simulink model "vhs_fpga_rx_to_sdram_time_share_agc_cfo"  (Simulink 7.1)
settings: Solver=FixedStepDiscrete  SolverMode=SingleTasking  StartTime=0.0  StopTime=inf  RelTol=1e-3
values from neighbouring files (symbols this model uses):
  N_FB_RX_frame = 390    [OFDM_Parameter.mat]
  Nfft = 64    [OFDM_Parameter.mat]
  Nguard = 16    [OFDM_Parameter.mat]
  Nofdm = 130    [OFDM_Parameter.mat]
  Nskip = 8    [OFDM_Parameter.mat]
undefined symbols (not defined in the file or in its folder): Fs, Sincos_Bits, Sincos_Len, Theta_Bits
libraries: xbsIndex_r4 x366, vhsadac_common_ob_fpgalib_v1_2_0 x18, misc_tools_fpgalib_v1_0_0 x6, rffe_fpgalib_v1_1_0 x1, rtdex_fpgalib_v1_1_0 x1
(part 2 of 5)

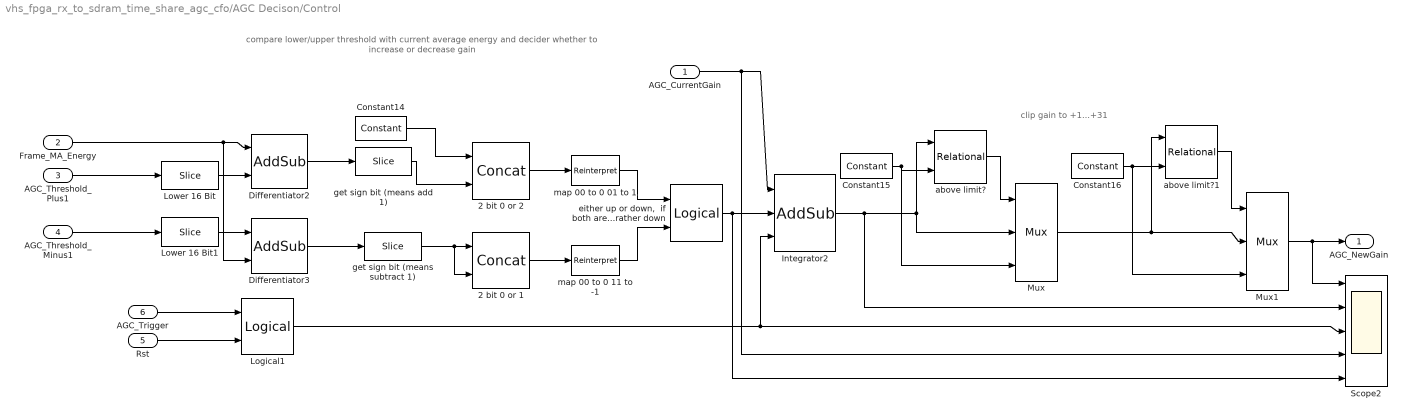
== system vhs_fpga_rx_to_sdram_time_share_agc_cfo/AGC Decison/Control ==
  note: compare lower/upper threshold with current average energy
      | and decider whether to increase or decrease gain
  note: clip gain to +1...+31
  AGC_CurrentGain : Inport
  Frame_MA_Energy : Inport  Port=2
  AGC_Threshold_Plus1 : Inport  Port=3
  AGC_Threshold_Minus1 : Inport  Port=4
  Rst : Inport  Port=5
  AGC_Trigger : Inport  Port=6
  2 bit 0 or 1 : xbsIndex_r4/Concat  num_inputs=2  dbl_ovrd=off  block_type=concat
      settings: block_version=10.1.3
  2 bit 0 or 2 : xbsIndex_r4/Concat  num_inputs=2  dbl_ovrd=off  block_type=concat
      settings: block_version=10.1.3
  Constant14 : xbsIndex_r4/Constant  arith_type=Unsigned  const=0  n_bits=1  bin_pt=0  explicit_period=on  period=5  equ=P=C  opselect=C  inp2=PCIN>>17  opr=+  inp1=P  carry=CIN  dbl_ovrd=off  block_type=constant
  Constant15 : xbsIndex_r4/Constant  arith_type=Signed (2's comp)  const=31  n_bits=32  bin_pt=0  explicit_period=on  period=5  equ=P=C  opselect=C  inp2=PCIN>>17  opr=+  inp1=P  carry=CIN  dbl_ovrd=off  block_type=constant
  Constant16 : xbsIndex_r4/Constant  arith_type=Signed (2's comp)  const=1  n_bits=32  bin_pt=0  explicit_period=on  period=5  equ=P=C  opselect=C  inp2=PCIN>>17  opr=+  inp1=P  carry=CIN  dbl_ovrd=off  block_type=constant
  Differentiator2 : xbsIndex_r4/AddSub  mode=Subtraction  use_carryin=off  use_carryout=off  en=off  latency=0  precision=Full  arith_type=Unsigned  n_bits=16  bin_pt=14  quantization=Truncate  overflow=Wrap  dbl_ovrd=off  use_behavioral_HDL=off  pipelined=off  use_rpm=on  hw_selection=Fabric  block_type=addsub
      settings: block_version=10.1.3
  Differentiator3 : xbsIndex_r4/AddSub  mode=Subtraction  use_carryin=off  use_carryout=off  en=off  latency=0  precision=Full  arith_type=Unsigned  n_bits=16  bin_pt=14  quantization=Truncate  overflow=Wrap  dbl_ovrd=off  use_behavioral_HDL=off  pipelined=off  use_rpm=on  hw_selection=Fabric  block_type=addsub
      settings: block_version=10.1.3
  Integrator2 : xbsIndex_r4/AddSub  mode=Addition  use_carryin=off  use_carryout=off  en=on  latency=1  precision=User Defined  arith_type="Signed  (2's comp)"  n_bits=32  bin_pt=0  quantization=Truncate  overflow=Saturate  dbl_ovrd=off  use_behavioral_HDL=off  pipelined=off  use_rpm=on  hw_selection=Fabric  block_type=addsub
      settings: block_version=10.1.3
  Logical1 : xbsIndex_r4/Logical  logical_function=OR  inputs=2  en=off  latency=0  precision=Full  arith_type=Unsigned  n_bits=16  bin_pt=0  align_bp=on  dbl_ovrd=off  block_type=logical
  Lower 16 Bit : xbsIndex_r4/Slice  nbits=16  boolean_output=off  mode=Upper Bit Location + Width  bit1=-16  base1=MSB of Input  bit0=0  base0=LSB of Input  dbl_ovrd=off  block_type=slice
      settings: infoedit="Extracts a given range of bits from each input sample and presents it at the output.  The output type is ordinarily unsigned with binary point at zero, but can be Boolean when the slice is one bit wide.<P><P>Hardware notes: In hardware this block costs nothing."  block_version=10.1.3
  Lower 16 Bit1 : xbsIndex_r4/Slice  nbits=16  boolean_output=off  mode=Upper Bit Location + Width  bit1=-16  base1=MSB of Input  bit0=0  base0=LSB of Input  dbl_ovrd=off  block_type=slice
      settings: infoedit="Extracts a given range of bits from each input sample and presents it at the output.  The output type is ordinarily unsigned with binary point at zero, but can be Boolean when the slice is one bit wide.<P><P>Hardware notes: In hardware this block costs nothing."  block_version=10.1.3
  Mux : xbsIndex_r4/Mux  inputs=2  en=off  latency=0  precision=Full  arith_type=Unsigned  n_bits=16  bin_pt=14  quantization=Truncate  overflow=Wrap  dbl_ovrd=off  block_type=mux
  Mux1 : xbsIndex_r4/Mux  inputs=2  en=off  latency=0  precision=Full  arith_type=Unsigned  n_bits=16  bin_pt=14  quantization=Truncate  overflow=Wrap  dbl_ovrd=off  block_type=mux
  Scope2 : Scope  NumInputPorts=5
      settings: TimeRange=369.8207656148967  YMin=1~0~0~0~0  YMax=2~2~1~15~1  SaveName=ScopeData2  MaxDataPoints=500000
  above limit? : xbsIndex_r4/Relational  mode=a>=b  en=off  latency=0  dbl_ovrd=off  block_type=relational
      settings: block_version=10.1.3
  above limit?1 : xbsIndex_r4/Relational  mode=a<=b  en=off  latency=0  dbl_ovrd=off  block_type=relational
      settings: block_version=10.1.3
  "either up or down,  if both are set, then rather down" : xbsIndex_r4/Logical  logical_function=OR  inputs=2  en=off  latency=0  precision=Full  arith_type=Unsigned  n_bits=16  bin_pt=0  align_bp=on  dbl_ovrd=off  block_type=logical
  get sign bit (means add 1) : xbsIndex_r4/Slice  nbits=1  boolean_output=off  mode=Upper Bit Location + Width  bit1=0  base1=MSB of Input  bit0=0  base0=LSB of Input  dbl_ovrd=off  block_type=slice
      settings: infoedit="Extracts a given range of bits from each input sample and presents it at the output.  The output type is ordinarily unsigned with binary point at zero, but can be Boolean when the slice is one bit wide.<P><P>Hardware notes: In hardware this block costs nothing."  block_version=10.1.3
  get sign bit (means subtract 1) : xbsIndex_r4/Slice  nbits=1  boolean_output=off  mode=Upper Bit Location + Width  bit1=0  base1=MSB of Input  bit0=0  base0=LSB of Input  dbl_ovrd=off  block_type=slice
      settings: infoedit="Extracts a given range of bits from each input sample and presents it at the output.  The output type is ordinarily unsigned with binary point at zero, but can be Boolean when the slice is one bit wide.<P><P>Hardware notes: In hardware this block costs nothing."  block_version=10.1.3
  map 00 to 0 01 to 1 : xbsIndex_r4/Reinterpret  force_arith_type=on  arith_type="Signed  (2's comp)"  force_bin_pt=on  bin_pt=0  block_type=reinterpret
      settings: infoedit="Changes signal type without altering the binary representation.   You can changed the signal between signed and unsigned, and relocate the binary point.<P><P>Hardware notes: In hardware this block costs nothing.<P><P>Example:  Suppose the input is 6 bits wide, signed, with 2 fractional bits, and the output is forced to unsigned with 0 fractional bits.  Then an input of -2.0 (1110.00 in binary 2's complement) becomes an output of 56 (111000 in binary)."  block_version=10.1.3
  map 00 to 0 11 to -1 : xbsIndex_r4/Reinterpret  force_arith_type=on  arith_type="Signed  (2's comp)"  force_bin_pt=on  bin_pt=0  block_type=reinterpret
      settings: infoedit="Changes signal type without altering the binary representation.   You can changed the signal between signed and unsigned, and relocate the binary point.<P><P>Hardware notes: In hardware this block costs nothing.<P><P>Example:  Suppose the input is 6 bits wide, signed, with 2 fractional bits, and the output is forced to unsigned with 0 fractional bits.  Then an input of -2.0 (1110.00 in binary 2's complement) becomes an output of 56 (111000 in binary)."  block_version=10.1.3
  AGC_NewGain : Outport
  wires:
  Lower 16 Bit/1 -> Differentiator2/2
  Frame_MA_Energy/1 -> Differentiator3/2, Differentiator2/1
  Lower 16 Bit1/1 -> Differentiator3/1
  Differentiator2/1 -> get sign bit (means add 1)/1
  Differentiator3/1 -> get sign bit (means subtract 1)/1
  get sign bit (means subtract 1)/1 -> 2 bit 0 or 1/1, 2 bit 0 or 1/2
  2 bit 0 or 1/1 -> map 00 to 0 11 to -1/1
  get sign bit (means add 1)/1 -> 2 bit 0 or 2/2
  Constant14/1 -> 2 bit 0 or 2/1
  2 bit 0 or 2/1 -> map 00 to 0 01 to 1/1
  map 00 to 0 01 to 1/1 -> "either up or down,  if both are set, then rather down"/1
  map 00 to 0 11 to -1/1 -> "either up or down,  if both are set, then rather down"/2
  "either up or down,  if both are set, then rather down"/1 -> Integrator2/2, Scope2/5
  Constant15/1 -> above limit?/2, Mux/3
  above limit?/1 -> Mux/1
  Integrator2/1 -> above limit?/1, Mux/2, Scope2/2
  Constant16/1 -> above limit?1/2, Mux1/3
  above limit?1/1 -> Mux1/1
  Mux1/1 -> Scope2/1, AGC_NewGain/1
  Mux/1 -> Mux1/2, above limit?1/1
  AGC_CurrentGain/1 -> Scope2/4, Integrator2/1
  AGC_Trigger/1 -> Logical1/1
  Logical1/1 -> Integrator2/3, Scope2/3
  AGC_Threshold_Plus1/1 -> Lower 16 Bit/1
  AGC_Threshold_Minus1/1 -> Lower 16 Bit1/1
  Rst/1 -> Logical1/2

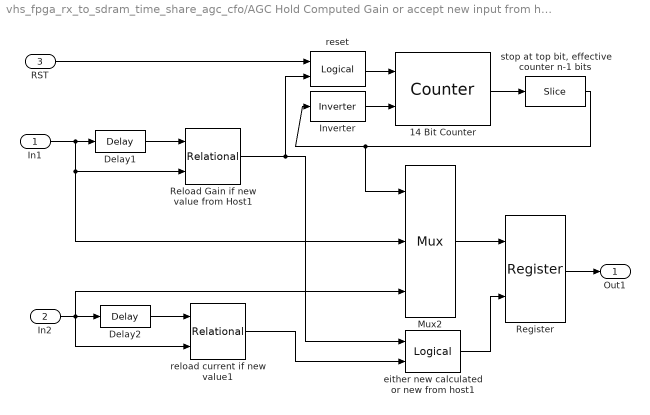
== system vhs_fpga_rx_to_sdram_time_share_agc_cfo/AGC Hold Computed Gain or accept new input from host ==
  In1 : Inport
  In2 : Inport  Port=2
  RST : Inport  Port=3
  14 Bit Counter : xbsIndex_r4/Counter  cnt_type=Free Running  cnt_to=Inf  operation=Up  start_count=0  cnt_by_val=1  arith_type=Unsigned  n_bits=14  bin_pt=0  load_pin=off  rst=on  en=on  explicit_period=off  period=1  dbl_ovrd=off  use_behavioral_HDL=off  use_rpm=off  implementation=Fabric  block_type=counter
  Delay1 : xbsIndex_r4/Delay  en=off  latency=1  dbl_ovrd=off  reg_retiming=off  block_type=delay
  Delay2 : xbsIndex_r4/Delay  en=off  latency=1  dbl_ovrd=off  reg_retiming=off  block_type=delay
  Inverter : xbsIndex_r4/Inverter  en=off  latency=0  dbl_ovrd=off  block_type=inv
  Mux2 : xbsIndex_r4/Mux  inputs=2  en=off  latency=0  precision=Full  arith_type=Unsigned  n_bits=16  bin_pt=14  quantization=Truncate  overflow=Wrap  dbl_ovrd=off  block_type=mux
  Register : xbsIndex_r4/Register  init=12  rst=off  en=on  dbl_ovrd=off  block_type=register
  Reload Gain if new value from Host1 : xbsIndex_r4/Relational  mode=a!=b  en=off  latency=1  dbl_ovrd=off  block_type=relational
      settings: block_version=10.1.3
  either new calculated or new from host1 : xbsIndex_r4/Logical  logical_function=OR  inputs=2  en=off  latency=1  precision=Full  arith_type=Unsigned  n_bits=16  bin_pt=0  align_bp=on  dbl_ovrd=off  block_type=logical
  reload current if new value1 : xbsIndex_r4/Relational  mode=a!=b  en=off  latency=1  dbl_ovrd=off  block_type=relational
      settings: block_version=10.1.3
  reset : xbsIndex_r4/Logical  logical_function=OR  inputs=2  en=off  latency=0  precision=Full  arith_type=Unsigned  n_bits=16  bin_pt=0  align_bp=on  dbl_ovrd=off  block_type=logical
  "stop at top bit, effective counter n-1 bits" : xbsIndex_r4/Slice  nbits=1  boolean_output=on  mode=Upper Bit Location + Width  bit1=0  base1=MSB of Input  bit0=0  base0=LSB of Input  dbl_ovrd=off  block_type=slice
      settings: infoedit="Extracts a given range of bits from each input sample and presents it at the output.  The output type is ordinarily unsigned with binary point at zero, but can be Boolean when the slice is one bit wide.<P><P>Hardware notes: In hardware this block costs nothing."  block_version=10.1.3
  Out1 : Outport
  wires:
  Delay1/1 -> Reload Gain if new value from Host1/1
  Reload Gain if new value from Host1/1 -> either new calculated or new from host1/1, reset/2
  Mux2/1 -> Register/1
  In1/1 -> Delay1/1, Reload Gain if new value from Host1/2, Mux2/2
  either new calculated or new from host1/1 -> Register/2
  Delay2/1 -> reload current if new value1/1
  In2/1 -> Delay2/1, reload current if new value1/2, Mux2/3
  reload current if new value1/1 -> either new calculated or new from host1/2
  Register/1 -> Out1/1
  Inverter/1 -> 14 Bit Counter/2
  "stop at top bit, effective counter n-1 bits"/1 -> Inverter/1, Mux2/1
  14 Bit Counter/1 -> "stop at top bit, effective counter n-1 bits"/1
  reset/1 -> 14 Bit Counter/1
  RST/1 -> reset/1

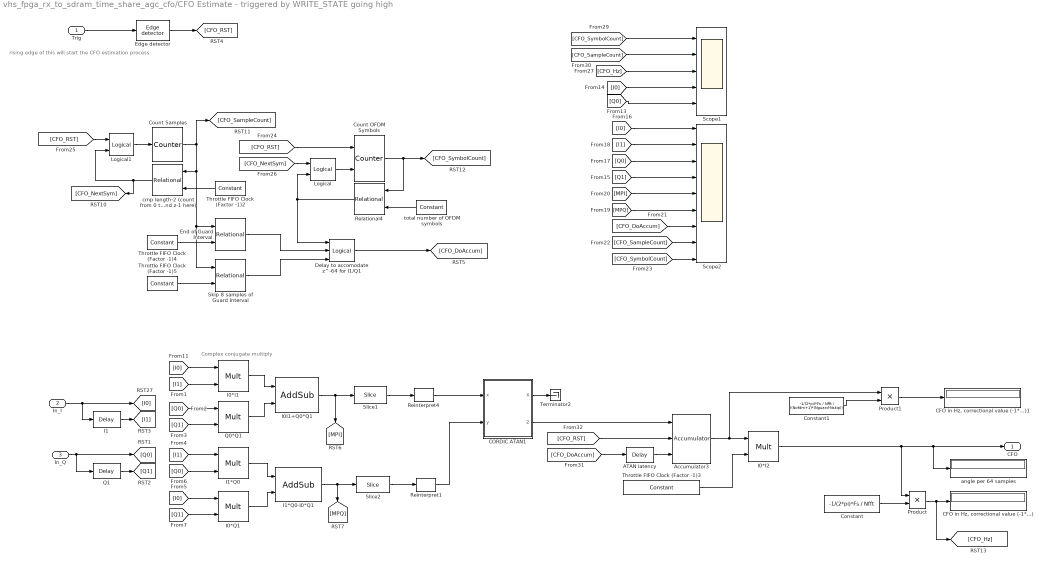
== system vhs_fpga_rx_to_sdram_time_share_agc_cfo/CFO Estimate - triggered by WRITE_STATE going high ==
  note: rising edge of this will start the
      | CFO estimation process
  note: Complex conjugate multiply
  Trig : Inport
  In_I : Inport  Port=2
  In_Q : Inport  Port=3
  ATAN latency : xbsIndex_r4/Delay  en=off  latency=16  dbl_ovrd=off  reg_retiming=off  block_type=delay
  Accumulator3 : xbsIndex_r4/Accumulator  operation=Add  n_bits=42  overflow=Saturate  scale=1  rst=on  hasbypass=off  en=on  dbl_ovrd=off  use_behavioral_HDL=on  implementation=Fabric  block_type=accum
      settings: infoedit="Adder or subtractor-based accumulator.   Output type and binary point position match the input.<P><P>Hardware notes: When \"Reinitialize with input 'b' on reset\" is selected, the accumulator is forced to run at the system rate even if the input 'b' is running at a slower rate."  block_version=10.1.3
  "CFO in Hz, correctional value (-1*...)" : Display
  "CFO in Hz, correctional value (-1*...)1" : Display
  CORDIC ATAN1 : Subsystem  mask(Xilinx CORDIC ATAN){stages=13, pe_nbits=32, pe_binpt=30, pipeline_x=ones(1,14), prev_stages=13, pipeline=[1  1  1  1  1  1  1  1  1  1  1  1  1]}
      mask prompts: stages "Number of Processing Elements (integer value starting from 1)"; pe_nbits "X, Y Data Width"; pe_binpt "X, Y Binary Point Position"; pipeline_x "Latency for each Processing Element [1 0 0 1]"; prev_stages "Previous Number of Stages"; pipeline "Previous Pipeline Values"
      mask help: A parallel implementation, circular vectoring mode CORDIC processor for performing rectangular-to-polar conversion. The number of iteration stages (and resultant output accuracy) and the processor arithmetic precision are controlled by the mask customization.
      mask init:
      | [bg,fg] = xlcmap('XBlock',0);
      | iPos = get_param(gcb,'Position');
      | iWidth=iPos(3)-iPos(1); iHeight=iPos(4)-iPos(2);
      | iCx=iWidth/2;
      | iCy=iHeight/2;
      | [logoX, logoY] = xlogo(iPos);
      | sav_gcb=gcb;
      | stages = round(sum(abs(stages)));
      | if (stages == 0)
      | 	stages = prev_stages;
      | end
      | x = zeros(1,stages);
      | pipe_size = max(size(pipeline_x));
      | if pipe_size >= stages
      | 	x(1,1:stages) = pipeline_x(1,1:stages);
      | else
      | 	x(1,1:pipe_size) = pipeline_x(1,1:pipe_size);
      | end
      | 
      | if (stages ~=prev_stages)
      | 	pipeline=x;
      | 	cordic_pe = find_system(gcb, 'lookUnderMasks', 'all', 'FollowLinks','on','masktype', 'CORDIC parallel PE');
      |     
      |   a=find_system(cordic_pe{1}, 'lookUnderMasks', 'all', 'FollowLinks','on','masktype', 'CORDIC iteration PE');
      |   for i= 2:length(a)
      |     for j=1:3
      | 	  delete_line(cordic_pe{1}, ['CORDIC PE' int2str(i-1) '/' int2str(j)], ['CORDIC PE' int2str(i) '/' int2str(j)]);
      |     end
      |   end
      |     if length(a)>0,
      |       delete_line(cordic_pe{1}, 'x/1', 'CORDIC PE1/1');
      |       delete_line(cordic_pe{1}, 'y/1', 'CORDIC PE1/2');
      |       delete_line(cordic_pe{1}, 'z/1', 'CORDIC PE1/3');
      |       delete_line(cordic_pe{1}, ['CORDIC PE' int2str(length(a)) '/1'],'X/1');
      |       delete_line(cordic_pe{1}, ['CORDIC PE' int2str(length(a)) '/2'],'Terminator/1');
      |       delete_line(cordic_pe{1}, ['CORDIC PE' int2str(length(a)) '/3'],'Z/1');
      |     elseif length(a)==0
      |       temp_port=get_param([cordic_pe{1} '/x'],'porthandles');
      |       temp_line=get_param(temp_port.Outport,'line');
      |       if temp_line>=0  delete_line(temp_line); end
      |       temp_port=get_param([cordic_pe{1} '/y'],'porthandles');
      |       temp_line=get_param(temp_port.Outport,'line');
      |       if temp_line>=0  delete_line(temp_line); end
      |       temp_port=get_param([cordic_pe{1} '/z'],'porthandles');
      |       temp_line=get_param(temp_port.Outport,'line');
      |       if temp_line>=0  delete_line(temp_line); end
      |     end
      | 
      |     for i=2:length(a)
      |       delete_block(a{i});
      |     end
      |     for i=2:stages,
      |         add_block([cordic_pe{1} '/CORDIC PE1'], [cordic_pe{1} '/CORDIC PE' int2str(i)], 'ii', int2str(i-1),'pe_nbits', 'pe_nbits','pe_binpt', 'pe_binpt','pipeline',['pipeline(1,' int2str(i) ')'],'position',[150+(i-1)*125, 70, 205+(i-1)*125, 130]);
      |     end
      | 
      |     for i= 2:stages,
      |       for j=1:3
      | 		add_line(cordic_pe{1}, ['CORDIC PE' int2str(i-1) '/' int2str(j)], ['CORDIC PE' int2str(i) '/' int2str(j)], 'autorouting', 'on');
      |       end
      |     end
      | 
      |     if stages==0
      |       add_line(cordic_pe{1}, 'x/1', 'X/1', 'autorouting', 'on');
      |       add_line(cordic_pe{1}, 'y/1', 'Terminator/1', 'autorouting', 'on');
      |       add_line(cordic_pe{1}, 'z/1', 'Z/1', 'autorouting', 'on');
      |     elseif stages>0
      |       add_line(cordic_pe{1}, 'x/1', 'CORDIC PE1/1', 'autorouting', 'on');
      |       add_line(cordic_pe{1}, 'y/1', 'CORDIC PE1/2', 'autorouting', 'on');
      |       add_line(cordic_pe{1}, 'z/1', 'CORDIC PE1/3', 'autorouting', 'on');
      | 
      |       set_param([cordic_pe{1} '/' 'X'], 'Position', [150+stages*125, 72, 180+stages*125, 86]);
      |       set_param([cordic_pe{1} '/' 'Terminator'], 'Position', [210+stages*125, 92, 225+stages*125, 108]);
      |       set_param([cordic_pe{1} '/' 'Z'], 'Position', [240+stages*125, 113, 270+stages*125, 127]);
      | 
      |       add_line(cordic_pe{1}, ['CORDIC PE' int2str(stages) '/1'], 'X/1', 'autorouting', 'on');
      |       add_line(cordic_pe{1}, ['CORDIC PE' int2str(stages) '/2'], 'Terminator/1', 'autorouting', 'on');
      |       add_line(cordic_pe{1}, ['CORDIC PE' int2str(stages) '/3'],'Z/1', 'autorouting', 'on');
      | 
      |       % force a "compile" of the constituent constant blocks to
      |       % workaround a data propagation problem
      |       find_system(cordic_pe{1}, 'lookUnderMasks', 'all', 'FollowLinks', 'on', 'MaskType','Xilinx Constant Block');
      |   end
      | 	set_param(sav_gcb, 'prev_stages', int2str(stages));
      | 	set_param(sav_gcb, 'pipeline', [ '[' int2str(x) ']']);
      | else
      | 	if (sum(pipeline~=x))
      | 		set_param(gcb, 'pipeline', [ '[' int2str(x) ']']);
      | 	end
      | end
      | str = sprintf('-%d',sum(x) + 3);
      settings: CopyFcn=set_param(gcb, 'MaskSelfModifiable', 'on', 'LinkStatus', 'none');
      mask Help: eval('');xlDoc('-book','sysgen','-topic','CORDIC_ATAN');
      mask Display:
      | patch([0 iWidth iWidth 0],[0 0 iHeight iHeight] , bg);
      | patch(logoX,logoY , fg);
      | text(iCx-6,iCy,'z');
      | text(iCx,iCy+4,str);
      | port_label('input',1,'x');
      | port_label('input',2,'y');
      | port_label('output',1,'mag');
      | port_label('output',2,'atan');
      | plot([0 0 iWidth iWidth 0], [0 iHeight iHeight 0 0]);
  Constant : Constant  Value=-1/(2*pi)*Fs / Nfft  OutDataType=sfix(16)  OutScaling=2^0  SampleTime=5
  Constant1 : Constant  Value=-1/(2*pi)*Fs / Nfft / ((Nofdm+1)*(Nguard-Nskip))  OutDataType=sfix(16)  OutScaling=2^0  SampleTime=5
  Count Samples : xbsIndex_r4/Counter  cnt_type=Free Running  cnt_to=Inf  operation=Up  start_count=0  cnt_by_val=1  arith_type=Unsigned  n_bits=7  bin_pt=0  load_pin=off  rst=on  en=off  explicit_period=on  period=5  dbl_ovrd=off  use_behavioral_HDL=off  use_rpm=off  implementation=Fabric  block_type=counter
      settings: block_version=VER_STRING_GOES_HERE
  Count OFDM Symbols : xbsIndex_r4/Counter  cnt_type=Free Running  cnt_to=Inf  operation=Up  start_count=0  cnt_by_val=1  arith_type=Unsigned  n_bits=8  bin_pt=0  load_pin=off  rst=on  en=on  explicit_period=on  period=5  dbl_ovrd=off  use_behavioral_HDL=off  use_rpm=off  implementation=Fabric  block_type=counter
      settings: block_version=VER_STRING_GOES_HERE
  Delay to accomodate z^-64 for I1/Q1 : xbsIndex_r4/Logical  logical_function=AND  inputs=3  en=off  latency=Nfft-3+1  precision=Full  arith_type=Unsigned  n_bits=16  bin_pt=0  align_bp=on  dbl_ovrd=off  block_type=logical
  Edge detector : misc_tools_fpgalib_v1_0_0/Edge detector  Tag=LYR_FPGA_MISC_EDGE_DETECTOR  Description=Lyrtech block  SystemSampleTime=-1  edge_detect=Rising  and_latency=0
  End of Guard Interval : xbsIndex_r4/Relational  mode=a<=b  en=off  latency=0  dbl_ovrd=off  block_type=relational
      settings: block_version=VER_STRING_GOES_HERE
  I0*I1 : xbsIndex_r4/Mult  precision=Full  arith_type="Signed  (2's comp)"  n_bits=16  bin_pt=14  quantization=Truncate  overflow=Wrap  en=off  latency=3  dbl_ovrd=off  use_behavioral_HDL=off  use_embedded=on  opt=Speed  optimum_pipeline=off  pipeline=on  use_rpm=on  placement_style=Triangular  block_type=mult
      settings: infoedit=Hardware notes: To use the internal pipeline stage of the dedicated multiplier you must select 'Pipeline for maximum performance'.  block_version=10.1.3
  I0*I2 : xbsIndex_r4/Mult  precision=User Defined  arith_type="Signed  (2's comp)"  n_bits=32  bin_pt=30  quantization=Truncate  overflow=Wrap  en=off  latency=3  dbl_ovrd=off  use_behavioral_HDL=off  use_embedded=on  opt=Speed  optimum_pipeline=off  pipeline=on  use_rpm=on  placement_style=Triangular  block_type=mult
      settings: infoedit=Hardware notes: To use the internal pipeline stage of the dedicated multiplier you must select 'Pipeline for maximum performance'.  block_version=10.1.3
  I0*Q1 : xbsIndex_r4/Mult  precision=Full  arith_type="Signed  (2's comp)"  n_bits=16  bin_pt=14  quantization=Truncate  overflow=Wrap  en=off  latency=3  dbl_ovrd=off  use_behavioral_HDL=off  use_embedded=on  opt=Speed  optimum_pipeline=off  pipeline=on  use_rpm=on  placement_style=Triangular  block_type=mult
      settings: infoedit=Hardware notes: To use the internal pipeline stage of the dedicated multiplier you must select 'Pipeline for maximum performance'.  block_version=10.1.3
  I0I1+Q0*Q1 : xbsIndex_r4/AddSub  mode=Addition  use_carryin=off  use_carryout=off  en=off  latency=1  precision=Full  arith_type=Unsigned  n_bits=16  bin_pt=14  quantization=Truncate  overflow=Wrap  dbl_ovrd=off  use_behavioral_HDL=off  pipelined=off  use_rpm=on  hw_selection=Fabric  block_type=addsub
      settings: block_version=10.1.3
  I1 : xbsIndex_r4/Delay  en=off  latency=Nfft  dbl_ovrd=off  reg_retiming=off  block_type=delay
  I1*Q0 : xbsIndex_r4/Mult  precision=Full  arith_type="Signed  (2's comp)"  n_bits=16  bin_pt=14  quantization=Truncate  overflow=Wrap  en=off  latency=3  dbl_ovrd=off  use_behavioral_HDL=off  use_embedded=on  opt=Speed  optimum_pipeline=off  pipeline=on  use_rpm=on  placement_style=Triangular  block_type=mult
      settings: infoedit=Hardware notes: To use the internal pipeline stage of the dedicated multiplier you must select 'Pipeline for maximum performance'.  block_version=10.1.3
  I1*Q0-I0*Q1 : xbsIndex_r4/AddSub  mode=Subtraction  use_carryin=off  use_carryout=off  en=off  latency=1  precision=Full  arith_type=Unsigned  n_bits=16  bin_pt=14  quantization=Truncate  overflow=Wrap  dbl_ovrd=off  use_behavioral_HDL=off  pipelined=off  use_rpm=on  hw_selection=Fabric  block_type=addsub
      settings: block_version=10.1.3
  Logical : xbsIndex_r4/Logical  logical_function=AND  inputs=2  en=off  latency=0  precision=Full  arith_type=Unsigned  n_bits=16  bin_pt=0  align_bp=on  dbl_ovrd=off  block_type=logical
  Logical1 : xbsIndex_r4/Logical  logical_function=OR  inputs=2  en=off  latency=0  precision=Full  arith_type=Unsigned  n_bits=16  bin_pt=0  align_bp=on  dbl_ovrd=off  block_type=logical
  Product : Product  OutDataType=sfix(16)  OutScaling=2^0  RndMeth=Zero
  Product1 : Product  OutDataType=sfix(16)  OutScaling=2^0  RndMeth=Zero
  Q0*Q1 : xbsIndex_r4/Mult  precision=Full  arith_type="Signed  (2's comp)"  n_bits=16  bin_pt=14  quantization=Truncate  overflow=Wrap  en=off  latency=3  dbl_ovrd=off  use_behavioral_HDL=off  use_embedded=on  opt=Speed  optimum_pipeline=off  pipeline=on  use_rpm=on  placement_style=Triangular  block_type=mult
      settings: infoedit=Hardware notes: To use the internal pipeline stage of the dedicated multiplier you must select 'Pipeline for maximum performance'.  block_version=10.1.3
  Q1 : xbsIndex_r4/Delay  en=off  latency=Nfft  dbl_ovrd=off  reg_retiming=off  block_type=delay
  Reinterpret1 : xbsIndex_r4/Reinterpret  force_arith_type=on  arith_type="Signed  (2's comp)"  force_bin_pt=on  bin_pt=30  block_type=reinterpret
      settings: infoedit="Changes signal type without altering the binary representation.   You can changed the signal between signed and unsigned, and relocate the binary point.<P><P>Hardware notes: In hardware this block costs nothing.<P><P>Example:  Suppose the input is 6 bits wide, signed, with 2 fractional bits, and the output is forced to unsigned with 0 fractional bits.  Then an input of -2.0 (1110.00 in binary 2's complement) becomes an output of 56 (111000 in binary)."  block_version=10.1.3
  Reinterpret4 : xbsIndex_r4/Reinterpret  force_arith_type=on  arith_type="Signed  (2's comp)"  force_bin_pt=on  bin_pt=30  block_type=reinterpret
      settings: infoedit="Changes signal type without altering the binary representation.   You can changed the signal between signed and unsigned, and relocate the binary point.<P><P>Hardware notes: In hardware this block costs nothing.<P><P>Example:  Suppose the input is 6 bits wide, signed, with 2 fractional bits, and the output is forced to unsigned with 0 fractional bits.  Then an input of -2.0 (1110.00 in binary 2's complement) becomes an output of 56 (111000 in binary)."  block_version=10.1.3
  Relational4 : xbsIndex_r4/Relational  Orientation=left  mode=a<b  en=off  latency=0  dbl_ovrd=off  block_type=relational
      settings: block_version=VER_STRING_GOES_HERE
  Scope1 : Scope  NumInputPorts=5
      settings: YMin=-5~-5~-5~-5~-5  YMax=5~5~5~5~5  SaveName=ScopeData8  MaxDataPoints=500000
  Scope2 : Scope  NumInputPorts=9
      settings: YMin=-5~-5~-5~-5~-5~-5~-5~-5~-5  YMax=5~5~5~5~5~5~5~5~5  MaxDataPoints=500000
  Skip 8 samples of Guard Interval : xbsIndex_r4/Relational  mode=a>b  en=off  latency=0  dbl_ovrd=off  block_type=relational
      settings: block_version=VER_STRING_GOES_HERE
  Slice1 : xbsIndex_r4/Slice  nbits=32  boolean_output=off  mode=Upper Bit Location + Width  bit1=0  base1=MSB of Input  bit0=0  base0=LSB of Input  dbl_ovrd=off  block_type=slice
      settings: infoedit="Extracts a given range of bits from each input sample and presents it at the output.  The output type is ordinarily unsigned with binary point at zero, but can be Boolean when the slice is one bit wide.<P><P>Hardware notes: In hardware this block costs nothing."  block_version=10.1.3
  Slice2 : xbsIndex_r4/Slice  nbits=32  boolean_output=off  mode=Upper Bit Location + Width  bit1=0  base1=MSB of Input  bit0=0  base0=LSB of Input  dbl_ovrd=off  block_type=slice
      settings: infoedit="Extracts a given range of bits from each input sample and presents it at the output.  The output type is ordinarily unsigned with binary point at zero, but can be Boolean when the slice is one bit wide.<P><P>Hardware notes: In hardware this block costs nothing."  block_version=10.1.3
  Terminator2 : Terminator
  Throttle FIFO Clock (Factor -1)2 : xbsIndex_r4/Constant  Orientation=left  arith_type=Unsigned  const=Nfft+Nguard-2  n_bits=7  bin_pt=0  explicit_period=on  period=5  equ=P=C  opselect=C  inp2=PCIN>>17  opr=+  inp1=P  carry=CIN  dbl_ovrd=off  block_type=constant
  Throttle FIFO Clock (Factor -1)3 : xbsIndex_r4/Constant  arith_type=Unsigned  const=1/((Nofdm+1)*(Nguard-Nskip))  n_bits=33  bin_pt=31  explicit_period=on  period=5  equ=P=C  opselect=C  inp2=PCIN>>17  opr=+  inp1=P  carry=CIN  dbl_ovrd=off  block_type=constant
  Throttle FIFO Clock (Factor -1)4 : xbsIndex_r4/Constant  arith_type=Unsigned  const=Nguard  n_bits=7  bin_pt=0  explicit_period=on  period=5  equ=P=C  opselect=C  inp2=PCIN>>17  opr=+  inp1=P  carry=CIN  dbl_ovrd=off  block_type=constant
  Throttle FIFO Clock (Factor -1)5 : xbsIndex_r4/Constant  arith_type=Unsigned  const=Nskip  n_bits=7  bin_pt=0  explicit_period=on  period=5  equ=P=C  opselect=C  inp2=PCIN>>17  opr=+  inp1=P  carry=CIN  dbl_ovrd=off  block_type=constant
  angle per 64 samples : Display
  cmp length-2 (count from 0 to len-1 and z-1 here) : xbsIndex_r4/Relational  Orientation=left  mode=a=b  en=off  latency=1  dbl_ovrd=off  block_type=relational
      settings: block_version=VER_STRING_GOES_HERE
  total number of OFDM symbols : xbsIndex_r4/Constant  Orientation=left  arith_type=Unsigned  const=(Nofdm+1)  n_bits=8  bin_pt=0  explicit_period=on  period=5  equ=P=C  opselect=C  inp2=PCIN>>17  opr=+  inp1=P  carry=CIN  dbl_ovrd=off  block_type=constant
  CFO : Outport
  wires:
  Trig/1 -> Edge detector/1
  Edge detector/1 -> [CFO_RST]
  Count OFDM Symbols/1 -> Relational4/1, [CFO_SymbolCount]
  total number of OFDM symbols/1 -> Relational4/2
  In_I/1 -> I1/1, [I0]
  In_Q/1 -> Q1/1, [Q0]
  I1/1 -> [I1]
  I0*I1/1 -> I0I1+Q0*Q1/1
  Q0*Q1/1 -> I0I1+Q0*Q1/2
  I1*Q0/1 -> I1*Q0-I0*Q1/1
  I0*Q1/1 -> I1*Q0-I0*Q1/2
  Q1/1 -> [Q1]
  [I0] -> I0*I1/1
  [I1] -> I0*I1/2
  [Q0] -> Q0*Q1/1
  [Q1] -> Q0*Q1/2
  [I1] -> I1*Q0/1
  [Q0] -> I1*Q0/2
  [I0] -> I0*Q1/1
  [Q1] -> I0*Q1/2
  I0I1+Q0*Q1/1 -> Slice1/1, [MPI]
  Slice1/1 -> Reinterpret4/1
  Slice2/1 -> Reinterpret1/1
  I1*Q0-I0*Q1/1 -> Slice2/1, [MPQ]
  Reinterpret4/1 -> CORDIC ATAN1/1(x)
  Reinterpret1/1 -> CORDIC ATAN1/2(y)
  [I0] -> Scope2/1
  [I1] -> Scope2/2
  [Q0] -> Scope2/3
  [Q1] -> Scope2/4
  [MPI] -> Scope2/5
  [MPQ] -> Scope2/6
  [CFO_DoAccum] -> Scope2/7
  Logical/1 -> Count OFDM Symbols/2
  Relational4/1 -> Logical/2, Delay to accomodate z^-64 for I1/Q1/1
  [CFO_RST] -> Count OFDM Symbols/1
  Throttle FIFO Clock (Factor -1)2/1 -> cmp length-2 (count from 0 to len-1 and z-1 here)/2
  Count Samples/1 -> [CFO_SampleCount], cmp length-2 (count from 0 to len-1 and z-1 here)/1, End of Guard Interval/1, Skip 8 samples of Guard Interval/1
  Logical1/1 -> Count Samples/1
  [CFO_RST] -> Logical1/1
  cmp length-2 (count from 0 to len-1 and z-1 here)/1 -> Logical1/2, [CFO_NextSym]
  [CFO_NextSym] -> Logical/1
  [CFO_SampleCount] -> Scope2/8
  [CFO_SymbolCount] -> Scope2/9
  Throttle FIFO Clock (Factor -1)4/1 -> End of Guard Interval/2
  Throttle FIFO Clock (Factor -1)5/1 -> Skip 8 samples of Guard Interval/2
  Delay to accomodate z^-64 for I1/Q1/1 -> [CFO_DoAccum]
  End of Guard Interval/1 -> Delay to accomodate z^-64 for I1/Q1/2
  Skip 8 samples of Guard Interval/1 -> Delay to accomodate z^-64 for I1/Q1/3
  Product/1 -> "CFO in Hz, correctional value (-1*...)"/1, [CFO_Hz]
  Constant/1 -> Product/2
  [CFO_SymbolCount] -> Scope1/1
  [CFO_SampleCount] -> Scope1/2
  [CFO_RST] -> Accumulator3/2
  [CFO_DoAccum] -> ATAN latency/1
  CORDIC ATAN1/1(X) -> Terminator2/1
  ATAN latency/1 -> Accumulator3/3
  CORDIC ATAN1/2(Z) -> Accumulator3/1
  Accumulator3/1 -> I0*I2/1, Product1/1
  I0*I2/1 -> CFO/1, angle per 64 samples/1, Product/1
  Throttle FIFO Clock (Factor -1)3/1 -> I0*I2/2
  Product1/1 -> "CFO in Hz, correctional value (-1*...)1"/1
  Constant1/1 -> Product1/2
  [CFO_Hz] -> Scope1/3
  [I0] -> Scope1/4
  [Q0] -> Scope1/5

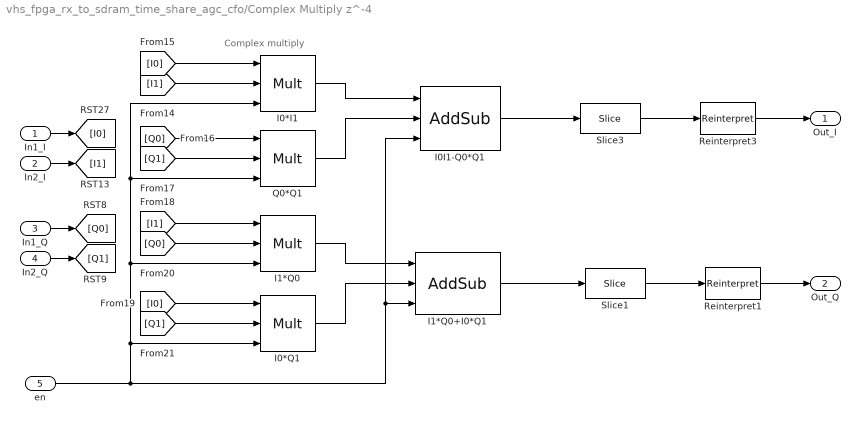
== system vhs_fpga_rx_to_sdram_time_share_agc_cfo/Complex Multiply z^-4 ==
  note: Complex multiply
  In1_I : Inport
  In2_I : Inport  Port=2
  In1_Q : Inport  Port=3
  In2_Q : Inport  Port=4
  en : Inport  Port=5
  I0*I1 : xbsIndex_r4/Mult  precision=Full  arith_type="Signed  (2's comp)"  n_bits=16  bin_pt=14  quantization=Truncate  overflow=Wrap  en=on  latency=3  dbl_ovrd=off  use_behavioral_HDL=off  use_embedded=on  opt=Speed  optimum_pipeline=off  pipeline=on  use_rpm=on  placement_style=Triangular  block_type=mult
      settings: infoedit=Hardware notes: To use the internal pipeline stage of the dedicated multiplier you must select 'Pipeline for maximum performance'.  block_version=10.1.3
  I0*Q1 : xbsIndex_r4/Mult  precision=Full  arith_type="Signed  (2's comp)"  n_bits=16  bin_pt=14  quantization=Truncate  overflow=Wrap  en=on  latency=3  dbl_ovrd=off  use_behavioral_HDL=off  use_embedded=on  opt=Speed  optimum_pipeline=off  pipeline=on  use_rpm=on  placement_style=Triangular  block_type=mult
      settings: infoedit=Hardware notes: To use the internal pipeline stage of the dedicated multiplier you must select 'Pipeline for maximum performance'.  block_version=10.1.3
  I0I1-Q0*Q1 : xbsIndex_r4/AddSub  mode=Subtraction  use_carryin=off  use_carryout=off  en=on  latency=1  precision=Full  arith_type=Unsigned  n_bits=16  bin_pt=14  quantization=Truncate  overflow=Wrap  dbl_ovrd=off  use_behavioral_HDL=off  pipelined=off  use_rpm=on  hw_selection=Fabric  block_type=addsub
      settings: block_version=10.1.3
  I1*Q0 : xbsIndex_r4/Mult  precision=Full  arith_type="Signed  (2's comp)"  n_bits=16  bin_pt=14  quantization=Truncate  overflow=Wrap  en=on  latency=3  dbl_ovrd=off  use_behavioral_HDL=off  use_embedded=on  opt=Speed  optimum_pipeline=off  pipeline=on  use_rpm=on  placement_style=Triangular  block_type=mult
      settings: infoedit=Hardware notes: To use the internal pipeline stage of the dedicated multiplier you must select 'Pipeline for maximum performance'.  block_version=10.1.3
  I1*Q0+I0*Q1 : xbsIndex_r4/AddSub  mode=Addition  use_carryin=off  use_carryout=off  en=on  latency=1  precision=Full  arith_type=Unsigned  n_bits=16  bin_pt=14  quantization=Truncate  overflow=Wrap  dbl_ovrd=off  use_behavioral_HDL=off  pipelined=off  use_rpm=on  hw_selection=Fabric  block_type=addsub
      settings: block_version=10.1.3
  Q0*Q1 : xbsIndex_r4/Mult  precision=Full  arith_type="Signed  (2's comp)"  n_bits=16  bin_pt=14  quantization=Truncate  overflow=Wrap  en=on  latency=3  dbl_ovrd=off  use_behavioral_HDL=off  use_embedded=on  opt=Speed  optimum_pipeline=off  pipeline=on  use_rpm=on  placement_style=Triangular  block_type=mult
      settings: infoedit=Hardware notes: To use the internal pipeline stage of the dedicated multiplier you must select 'Pipeline for maximum performance'.  block_version=10.1.3
  Reinterpret1 : xbsIndex_r4/Reinterpret  force_arith_type=on  arith_type="Signed  (2's comp)"  force_bin_pt=on  bin_pt=0  block_type=reinterpret
      settings: infoedit="Changes signal type without altering the binary representation.   You can changed the signal between signed and unsigned, and relocate the binary point.<P><P>Hardware notes: In hardware this block costs nothing.<P><P>Example:  Suppose the input is 6 bits wide, signed, with 2 fractional bits, and the output is forced to unsigned with 0 fractional bits.  Then an input of -2.0 (1110.00 in binary 2's complement) becomes an output of 56 (111000 in binary)."  block_version=10.1.3
  Reinterpret3 : xbsIndex_r4/Reinterpret  force_arith_type=on  arith_type="Signed  (2's comp)"  force_bin_pt=on  bin_pt=0  block_type=reinterpret
      settings: infoedit="Changes signal type without altering the binary representation.   You can changed the signal between signed and unsigned, and relocate the binary point.<P><P>Hardware notes: In hardware this block costs nothing.<P><P>Example:  Suppose the input is 6 bits wide, signed, with 2 fractional bits, and the output is forced to unsigned with 0 fractional bits.  Then an input of -2.0 (1110.00 in binary 2's complement) becomes an output of 56 (111000 in binary)."  block_version=10.1.3
  Slice1 : xbsIndex_r4/Slice  nbits=16  boolean_output=off  mode=Upper Bit Location + Width  bit1=0  base1=MSB of Input  bit0=0  base0=LSB of Input  dbl_ovrd=off  block_type=slice
      settings: infoedit="Extracts a given range of bits from each input sample and presents it at the output.  The output type is ordinarily unsigned with binary point at zero, but can be Boolean when the slice is one bit wide.<P><P>Hardware notes: In hardware this block costs nothing."  block_version=10.1.3
  Slice3 : xbsIndex_r4/Slice  nbits=16  boolean_output=off  mode=Upper Bit Location + Width  bit1=0  base1=MSB of Input  bit0=0  base0=LSB of Input  dbl_ovrd=off  block_type=slice
      settings: infoedit="Extracts a given range of bits from each input sample and presents it at the output.  The output type is ordinarily unsigned with binary point at zero, but can be Boolean when the slice is one bit wide.<P><P>Hardware notes: In hardware this block costs nothing."  block_version=10.1.3
  Out_I : Outport
  Out_Q : Outport  Port=2
  wires:
  I0*I1/1 -> I0I1-Q0*Q1/1
  Q0*Q1/1 -> I0I1-Q0*Q1/2
  I1*Q0/1 -> I1*Q0+I0*Q1/1
  I0*Q1/1 -> I1*Q0+I0*Q1/2
  [I0] -> I0*I1/1
  [I1] -> I0*I1/2
  [Q0] -> Q0*Q1/1
  [Q1] -> Q0*Q1/2
  [I1] -> I1*Q0/1
  [Q0] -> I1*Q0/2
  [I0] -> I0*Q1/1
  [Q1] -> I0*Q1/2
  I0I1-Q0*Q1/1 -> Slice3/1
  In1_I/1 -> [I0]
  In2_I/1 -> [I1]
  In1_Q/1 -> [Q0]
  In2_Q/1 -> [Q1]
  I1*Q0+I0*Q1/1 -> Slice1/1
  en/1 -> I0*Q1/3, I1*Q0/3, Q0*Q1/3, I0*I1/3, I1*Q0+I0*Q1/3, I0I1-Q0*Q1/3
  Slice3/1 -> Reinterpret3/1
  Reinterpret3/1 -> Out_I/1
  Slice1/1 -> Reinterpret1/1
  Reinterpret1/1 -> Out_Q/1

== system vhs_fpga_rx_to_sdram_time_share_agc_cfo/Delay 4, with Reset and Enable Flags ==
  In : Inport
  rst : Inport  Port=2
  en : Inport  Port=3
  Register{,1..3} (4 alike) : xbsIndex_r4/Register  init=0  rst=on  en=on  dbl_ovrd=off  block_type=register
  Out : Outport
  wires:
  Register/1 -> Register1/1
  Register1/1 -> Register2/1
  en/1 -> Register/3, Register1/3, Register2/3, Register3/3
  rst/1 -> Register1/2, Register2/2, Register3/2, Register/2
  In/1 -> Register/1
  Register3/1 -> Out/1
  Register2/1 -> Register3/1

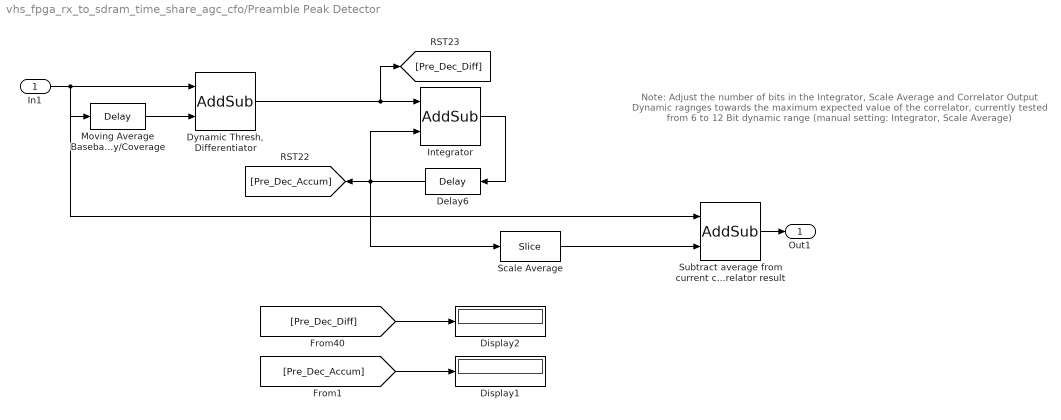
== system vhs_fpga_rx_to_sdram_time_share_agc_cfo/Preamble Peak Detector ==
  note: Note: Adjust the number of bits in the Integrator, Scale Average and Correlator Output Dynamic ragnges
      |  towards the maximum expected value of the correlator, currently tested from 6 to 12 Bit dynamic range
      |  (manual setting: Integrator, Scale Average)
  In1 : Inport
  Delay6 : xbsIndex_r4/Delay  Orientation=left  en=off  latency=1  dbl_ovrd=off  reg_retiming=off  block_type=delay
  Display1 : Display
  Display2 : Display
  "Dynamic Thresh, Differentiator" : xbsIndex_r4/AddSub  mode=Subtraction  use_carryin=off  use_carryout=off  en=off  latency=0  precision=Full  arith_type=Unsigned  n_bits=16  bin_pt=14  quantization=Truncate  overflow=Wrap  dbl_ovrd=off  use_behavioral_HDL=off  pipelined=off  use_rpm=on  hw_selection=Fabric  block_type=addsub
      settings: block_version=10.1.3
  Integrator : xbsIndex_r4/AddSub  mode=Addition  use_carryin=off  use_carryout=off  en=off  latency=0  precision=User Defined  arith_type="Signed  (2's comp)"  n_bits=23  bin_pt=0  quantization=Truncate  overflow=Saturate  dbl_ovrd=off  use_behavioral_HDL=off  pipelined=off  use_rpm=on  hw_selection=Fabric  block_type=addsub
      settings: block_version=10.1.3
  Moving Average Baseband (20MHz) Delay/Coverage : xbsIndex_r4/Delay  en=off  latency=32  dbl_ovrd=off  reg_retiming=off  block_type=delay
  Scale Average : xbsIndex_r4/Slice  nbits=16  boolean_output=off  mode=Upper Bit Location + Width  bit1=-7  base1=MSB of Input  bit0=0  base0=LSB of Input  dbl_ovrd=off  block_type=slice
      settings: infoedit="Extracts a given range of bits from each input sample and presents it at the output.  The output type is ordinarily unsigned with binary point at zero, but can be Boolean when the slice is one bit wide.<P><P>Hardware notes: In hardware this block costs nothing."  block_version=10.1.3
  Subtract average from current correlator result : xbsIndex_r4/AddSub  mode=Subtraction  use_carryin=off  use_carryout=off  en=off  latency=0  precision=Full  arith_type=Unsigned  n_bits=16  bin_pt=14  quantization=Truncate  overflow=Wrap  dbl_ovrd=off  use_behavioral_HDL=off  pipelined=off  use_rpm=on  hw_selection=Fabric  block_type=addsub
      settings: block_version=10.1.3
  Out1 : Outport
  wires:
  Moving Average Baseband (20MHz) Delay/Coverage/1 -> "Dynamic Thresh, Differentiator"/2
  "Dynamic Thresh, Differentiator"/1 -> Integrator/1, [Pre_Dec_Diff]
  Integrator/1 -> Delay6/1
  Delay6/1 -> Integrator/2, [Pre_Dec_Accum], Scale Average/1
  Scale Average/1 -> Subtract average from current correlator result/2
  In1/1 -> Moving Average Baseband (20MHz) Delay/Coverage/1, Subtract average from current correlator result/1, "Dynamic Thresh, Differentiator"/1
  Subtract average from current correlator result/1 -> Out1/1
  [Pre_Dec_Accum] -> Display1/1
  [Pre_Dec_Diff] -> Display2/1

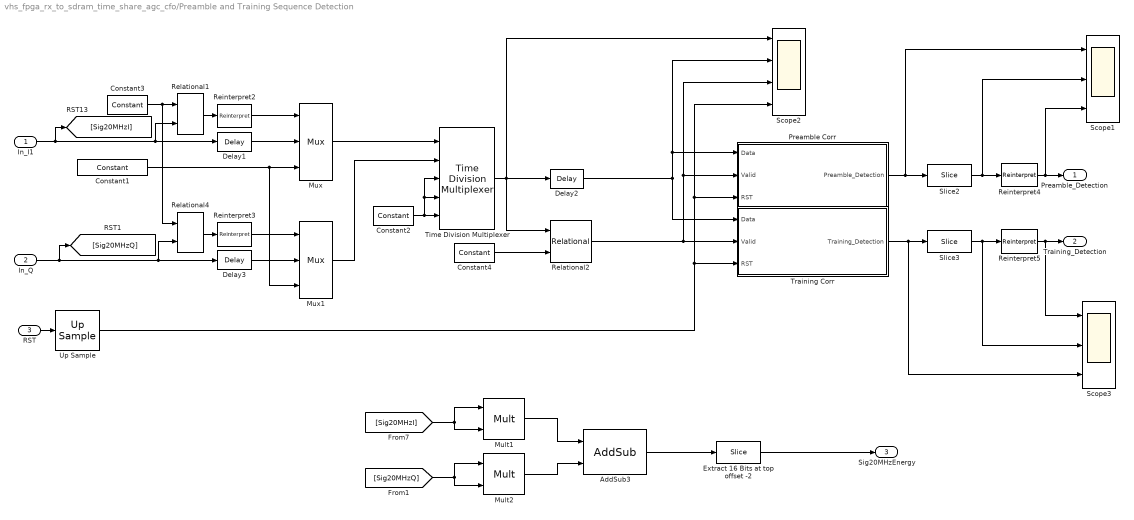
== system vhs_fpga_rx_to_sdram_time_share_agc_cfo/Preamble and Training Sequence Detection ==
  In_I1 : Inport  OutDataType=sfix(16)  OutScaling=2^0
  In_Q : Inport  Port=2  OutDataType=sfix(16)  OutScaling=2^0
  RST : Inport  Port=3  OutDataType=sfix(16)  OutScaling=2^0
  "   Extract 16 Bits at top offset -2" : xbsIndex_r4/Slice  nbits=16  boolean_output=off  mode=Upper Bit Location + Width  bit1=-2  base1=MSB of Input  bit0=0  base0=LSB of Input  dbl_ovrd=off  block_type=slice
      settings: infoedit="Extracts a given range of bits from each input sample and presents it at the output.  The output type is ordinarily unsigned with binary point at zero, but can be Boolean when the slice is one bit wide.<P><P>Hardware notes: In hardware this block costs nothing."  block_version=10.1.3
  AddSub3 : xbsIndex_r4/AddSub  mode=Addition  use_carryin=off  use_carryout=off  en=off  latency=1  precision=Full  arith_type=Unsigned  n_bits=16  bin_pt=14  quantization=Truncate  overflow=Wrap  dbl_ovrd=off  use_behavioral_HDL=off  pipelined=off  use_rpm=on  hw_selection=Fabric  block_type=addsub
      settings: block_version=10.1.3
  Constant1 : xbsIndex_r4/Constant  arith_type=Signed (2's comp)  const=1  n_bits=14  bin_pt=0  explicit_period=on  period=5  equ=P=C  opselect=C  inp2=PCIN>>17  opr=+  inp1=P  carry=CIN  dbl_ovrd=off  block_type=constant
  Constant2 : xbsIndex_r4/Constant  arith_type=Signed (2's comp)  const=0  n_bits=14  bin_pt=0  explicit_period=on  period=5  equ=P=C  opselect=C  inp2=PCIN>>17  opr=+  inp1=P  carry=CIN  dbl_ovrd=off  block_type=constant
  Constant3 : xbsIndex_r4/Constant  arith_type=Signed (2's comp)  const=0  n_bits=14  bin_pt=13  explicit_period=on  period=5  equ=P=C  opselect=C  inp2=PCIN>>17  opr=+  inp1=P  carry=CIN  dbl_ovrd=off  block_type=constant
  Constant4 : xbsIndex_r4/Constant  arith_type=Unsigned  const=0  n_bits=2  bin_pt=0  explicit_period=on  period=1  equ=P=C  opselect=C  inp2=PCIN>>17  opr=+  inp1=P  carry=CIN  dbl_ovrd=off  block_type=constant
  Delay1 : xbsIndex_r4/Delay  en=off  latency=1  dbl_ovrd=off  reg_retiming=off  block_type=delay
  Delay2 : xbsIndex_r4/Delay  en=off  latency=1  dbl_ovrd=off  reg_retiming=off  block_type=delay
  Delay3 : xbsIndex_r4/Delay  en=off  latency=1  dbl_ovrd=off  reg_retiming=off  block_type=delay
  Mult1 : xbsIndex_r4/Mult  precision=Full  arith_type="Signed  (2's comp)"  n_bits=16  bin_pt=14  quantization=Truncate  overflow=Wrap  en=off  latency=3  dbl_ovrd=off  use_behavioral_HDL=off  use_embedded=on  opt=Speed  optimum_pipeline=off  pipeline=on  use_rpm=on  placement_style=Triangular  block_type=mult
      settings: infoedit=Hardware notes: To use the internal pipeline stage of the dedicated multiplier you must select 'Pipeline for maximum performance'.  block_version=10.1.3
  Mult2 : xbsIndex_r4/Mult  precision=Full  arith_type="Signed  (2's comp)"  n_bits=16  bin_pt=14  quantization=Truncate  overflow=Wrap  en=off  latency=3  dbl_ovrd=off  use_behavioral_HDL=off  use_embedded=on  opt=Speed  optimum_pipeline=off  pipeline=on  use_rpm=on  placement_style=Triangular  block_type=mult
      settings: infoedit=Hardware notes: To use the internal pipeline stage of the dedicated multiplier you must select 'Pipeline for maximum performance'.  block_version=10.1.3
  Mux : xbsIndex_r4/Mux  inputs=2  en=off  latency=0  precision=Full  arith_type=Unsigned  n_bits=16  bin_pt=14  quantization=Truncate  overflow=Wrap  dbl_ovrd=off  block_type=mux
  Mux1 : xbsIndex_r4/Mux  inputs=2  en=off  latency=0  precision=Full  arith_type=Unsigned  n_bits=16  bin_pt=14  quantization=Truncate  overflow=Wrap  dbl_ovrd=off  block_type=mux
  Preamble Corr : Subsystem
  Reinterpret{2..5} (4 alike) : xbsIndex_r4/Reinterpret  force_arith_type=on  arith_type=Unsigned  force_bin_pt=on  bin_pt=0  block_type=reinterpret
      settings: infoedit="Changes signal type without altering the binary representation.   You can changed the signal between signed and unsigned, and relocate the binary point.<P><P>Hardware notes: In hardware this block costs nothing.<P><P>Example:  Suppose the input is 6 bits wide, signed, with 2 fractional bits, and the output is forced to unsigned with 0 fractional bits.  Then an input of -2.0 (1110.00 in binary 2's complement) becomes an output of 56 (111000 in binary)."  block_version=10.1.3
  Relational1 : xbsIndex_r4/Relational  mode=a=b  en=off  latency=1  dbl_ovrd=off  block_type=relational
      settings: block_version=10.1.3
  Relational2 : xbsIndex_r4/Relational  mode=a!=b  en=off  latency=1  dbl_ovrd=off  block_type=relational
      settings: block_version=10.1.3
  Relational4 : xbsIndex_r4/Relational  mode=a=b  en=off  latency=1  dbl_ovrd=off  block_type=relational
      settings: block_version=10.1.3
  Scope1 : Scope  NumInputPorts=3
      settings: YMin=-5~-5~-5  YMax=5~5~5  SaveName=ScopeData4  MaxDataPoints=500000  SampleInput=on
  Scope2 : Scope  NumInputPorts=4
      settings: YMin=-5~-5~-5~-5  YMax=5~5~5~5  SaveName=ScopeData3  MaxDataPoints=500000
  Scope3 : Scope  NumInputPorts=3
      settings: YMin=-5~-5~-5  YMax=5~5~5  SaveName=ScopeData5  MaxDataPoints=500000  SampleInput=on
  Slice2 : xbsIndex_r4/Slice  nbits=16  boolean_output=off  mode=Upper Bit Location + Width  bit1=-8  base1=MSB of Input  bit0=0  base0=LSB of Input  dbl_ovrd=off  block_type=slice
      settings: infoedit="Extracts a given range of bits from each input sample and presents it at the output.  The output type is ordinarily unsigned with binary point at zero, but can be Boolean when the slice is one bit wide.<P><P>Hardware notes: In hardware this block costs nothing."  block_version=10.1.3
  Slice3 : xbsIndex_r4/Slice  nbits=16  boolean_output=off  mode=Upper Bit Location + Width  bit1=-8  base1=MSB of Input  bit0=0  base0=LSB of Input  dbl_ovrd=off  block_type=slice
      settings: infoedit="Extracts a given range of bits from each input sample and presents it at the output.  The output type is ordinarily unsigned with binary point at zero, but can be Boolean when the slice is one bit wide.<P><P>Hardware notes: In hardware this block costs nothing."  block_version=10.1.3
  Time Division Multiplexer : xbsIndex_r4/Time Division Multiplexer  inputs=5  vin=off  dbl_ovrd=off  explicit_period=off  period=1  block_type=tdm
      settings: infoedit="Multiple inputs are sampled and  presented serially at the output."  block_version=10.1.3
  Training Corr : Subsystem
  Up Sample : xbsIndex_r4/Up Sample  sample_ratio=5  copy_samples=on  dbl_ovrd=off  block_type=usamp
      settings: infoedit="Up samples input data.  Inserted values  can be zeros or copies of the most recent input sample.<P><P>Hardware notes: No hardware is needed if inserted values are copies of the input sample; otherwise, a mux and single bit flip-flop are used."  block_version=10.1.3
  Preamble_Detection : Outport  OutDataType=sfix(16)  OutScaling=2^0
  Training_Detection : Outport  Port=2  OutDataType=sfix(16)  OutScaling=2^0
  Sig20MHzEnergy : Outport  Port=3  OutDataType=sfix(16)  OutScaling=2^0
  wires:
  Preamble Corr/1(Preamble_Detection) -> Slice2/1, Scope1/1
  Training Corr/1(Training_Detection) -> Slice3/1, Scope3/3
  Time Division Multiplexer/1 -> Delay2/1, Scope2/1, Relational2/1
  Constant2/1 -> Time Division Multiplexer/5, Time Division Multiplexer/3, Time Division Multiplexer/4
  In_Q/1 -> Relational4/2, Delay3/1, [Sig20MHzQ]
  In_I1/1 -> Relational1/2, Delay1/1, [Sig20MHzI]
  Constant4/1 -> Relational2/2
  RST/1 -> Up Sample/1
  Delay2/1 -> Training Corr/1(Data), Preamble Corr/1(Data), Scope2/2
  Up Sample/1 -> Training Corr/3(RST), Preamble Corr/3(RST), Scope2/4
  Relational2/1 -> Training Corr/2(Valid), Preamble Corr/2(Valid), Scope2/3
  Mux/1 -> Time Division Multiplexer/1
  Mux1/1 -> Time Division Multiplexer/2
  Constant1/1 -> Mux/3, Mux1/3
  Constant3/1 -> Relational1/1, Relational4/1
  Relational1/1 -> Reinterpret2/1
  Relational4/1 -> Reinterpret3/1
  Reinterpret2/1 -> Mux/1
  Reinterpret3/1 -> Mux1/1
  Delay1/1 -> Mux/2
  Delay3/1 -> Mux1/2
  Slice2/1 -> Reinterpret4/1, Scope1/2
  Slice3/1 -> Reinterpret5/1, Scope3/2
  Reinterpret4/1 -> Preamble_Detection/1, Scope1/3
  Reinterpret5/1 -> Training_Detection/1, Scope3/1
  [Sig20MHzI] -> Mult1/1, Mult1/2
  [Sig20MHzQ] -> Mult2/2, Mult2/1
  Mult1/1 -> AddSub3/1
  Mult2/1 -> AddSub3/2
  AddSub3/1 -> "   Extract 16 Bits at top offset -2"/1
  "   Extract 16 Bits at top offset -2"/1 -> Sig20MHzEnergy/1
